simulink model "Subject2"  (R2022b)
settings: Solver=VariableStepAuto  StartTime=0.0  StopTime=100  RelTol=1e-3
libraries: mpcadaslib x1
settings Model: Creator=ParkJunHo  LastModifiedBy=ParkJunHo

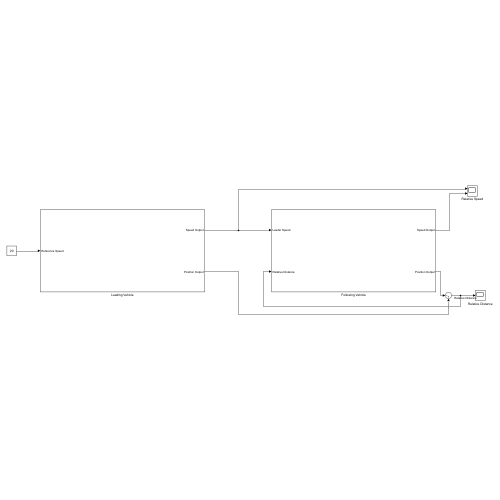
[thumbnail: Simulink's stored preview of the top-level diagram]
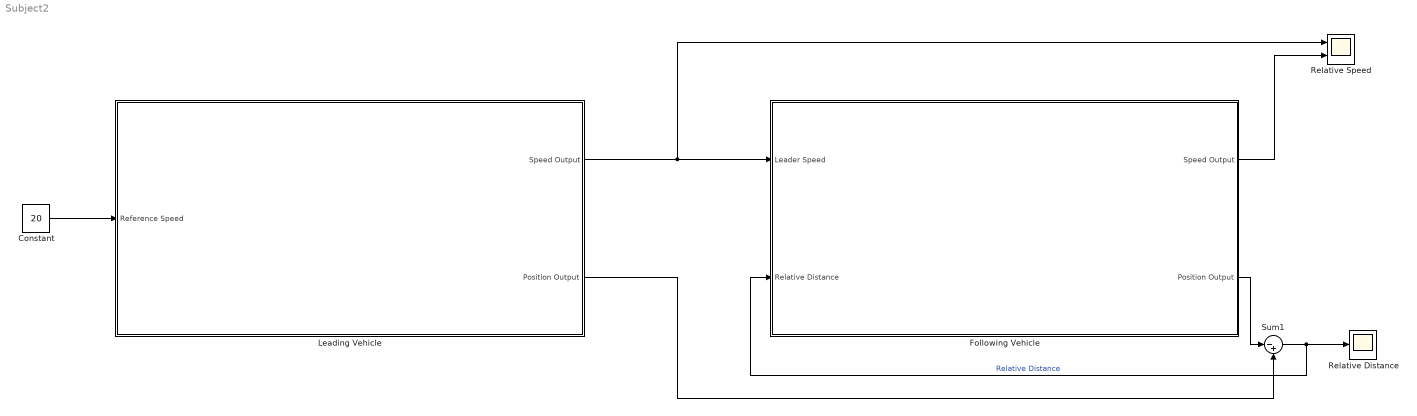
== system Subject2 ==
  Constant : Constant  Value=20
  Following Vehicle : Subsystem
  Leading Vehicle : Subsystem
  Relative Distance : Scope
  Relative Speed : Scope  NumInputPorts=2
  Sum1 : Sum  Inputs=|-+
  wires:
  Constant/1 -> Leading Vehicle/1(Reference Speed)
  Following Vehicle/1(Speed Output) -> Relative Speed/2
  Following Vehicle/2(Position Output) -> Sum1/1
  Leading Vehicle/1(Speed Output) -> Relative Speed/1, Following Vehicle/1(Leader Speed)
  Leading Vehicle/2(Position Output) -> Sum1/2
  Sum1/1 -> Following Vehicle/2(Relative Distance), Relative Distance/1  "Relative Distance"

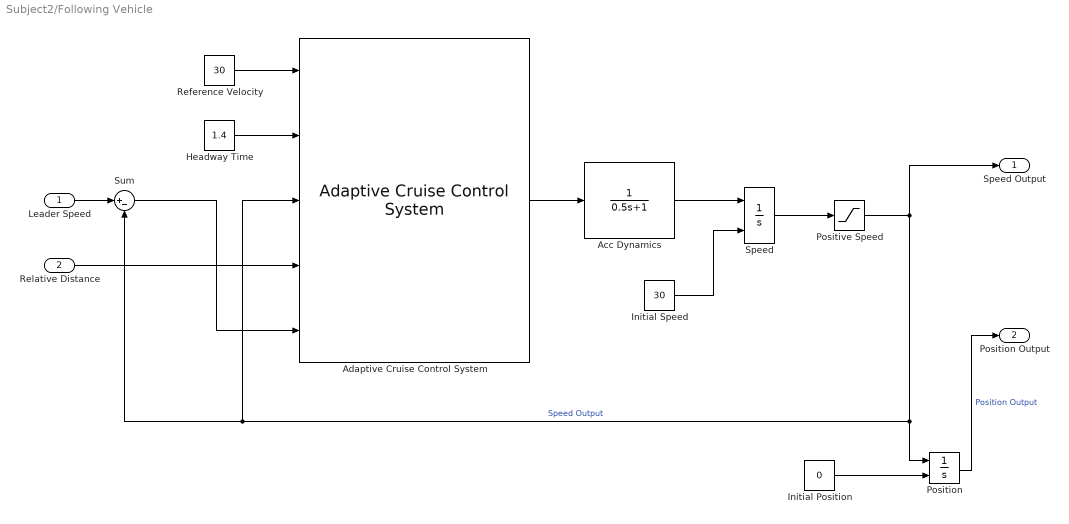
== system Subject2/Following Vehicle ==
  Leader Speed : Inport
  Relative Distance : Inport  Port=2
  Acc Dynamics : TransferFcn  Denominator=[0.5 1]
  Adaptive Cruise Control System : mpcadaslib/Adaptive Cruise Control System  EgoModel=tf(1,[0.5,1,0])  InitialEgoVelocity=30  DefaultSpacing=10  MaxVelocity=50  MinAcceleration=-3  amin_ext=off  MaxAcceleration=2  amax_ext=off  Ts=0.1  PredictionHorizon=300  ControllerBehavior=0.5  suboptimal=off  maxiter=10  datatypeopt=double  optmode=off  trackmode=off
      settings: LibrarySourceBlock=mpclib/Automated Driving/Adaptive Cruise Control System
  Headway Time : Constant  Value=1.4
  Initial Position : Constant  Value=0
  Initial Speed : Constant  Value=30
  Position : Integrator  InitialConditionSource=external
  Positive Speed : Saturate  UpperLimit=inf  LowerLimit=0
  Reference Velocity : Constant  Value=30
  Speed : Integrator  InitialConditionSource=external
  Sum : Sum  Inputs=|+-
  Speed Output : Outport
  Position Output : Outport  Port=2
  wires:
  Positive Speed/1 -> Speed Output/1, Position/1, Adaptive Cruise Control System/3, Sum/2  "Speed Output"
  Speed/1 -> Positive Speed/1
  Position/1 -> Position Output/1  "Position Output"
  Acc Dynamics/1 -> Speed/1
  Initial Position/1 -> Position/2
  Adaptive Cruise Control System/1 -> Acc Dynamics/1
  Initial Speed/1 -> Speed/2
  Leader Speed/1 -> Sum/1
  Sum/1 -> Adaptive Cruise Control System/5
  Relative Distance/1 -> Adaptive Cruise Control System/4
  Reference Velocity/1 -> Adaptive Cruise Control System/1
  Headway Time/1 -> Adaptive Cruise Control System/2

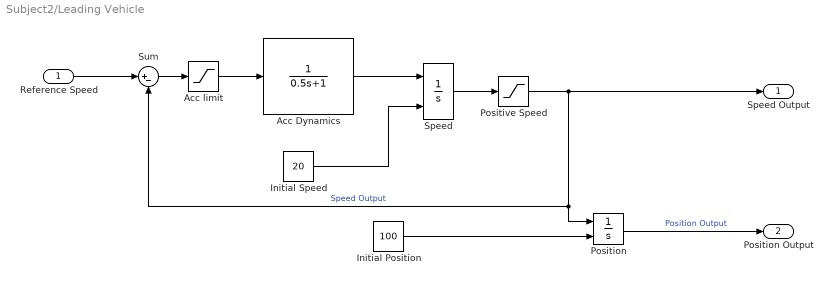
== system Subject2/Leading Vehicle ==
  Reference Speed : Inport
  Acc Dynamics : TransferFcn  Denominator=[0.5 1]
  Acc limit : Saturate  UpperLimit=2  LowerLimit=-3
  Initial Position : Constant  Value=100
  Initial Speed : Constant  Value=20
  Position : Integrator  InitialConditionSource=external
  Positive Speed : Saturate  UpperLimit=inf  LowerLimit=0
  Speed : Integrator  InitialConditionSource=external
  Sum : Sum  Inputs=|+-
  Speed Output : Outport
  Position Output : Outport  Port=2
  wires:
  Sum/1 -> Acc limit/1
  Positive Speed/1 -> Speed Output/1, Position/1, Sum/2  "Speed Output"
  Speed/1 -> Positive Speed/1
  Position/1 -> Position Output/1  "Position Output"
  Acc Dynamics/1 -> Speed/1
  Initial Position/1 -> Position/2
  Acc limit/1 -> Acc Dynamics/1
  Initial Speed/1 -> Speed/2
  Reference Speed/1 -> Sum/1
